simulink model "pi_client"  (R2019b)
settings: Solver=FixedStepAuto  StartTime=0.0  StopTime=10.0  RelTol=1e-3  EnableMultiTasking=on
values from neighbouring files (symbols this model uses):
  B = img(:,:,3)    [pi_client_script.m]
  Blank = R*0    [pi_client_script.m]
  G = img(:,:,2)    [pi_client_script.m]
  R = img(:,:,1)    [pi_client_script.m]
libraries: embdlinuxlib x1, raspberrypilib x1
settings Model: Creator=dhinojosac  LastModifiedBy=dhinojosac
settings SolverCC: PositivePriorityOrder=on
settings OptimizationCC: EnhancedBackFolding=on  PassReuseOutputArgsAs=Individual arguments  ZeroExternalMemoryAtStartup=off  ZeroInternalMemoryAtStartup=off  MaxStackSize=64  OptimizeBlockOrder=speed  DifferentSizesBufferReuse=on  OptimizationCustomize=off  EfficientTunableParamExpr=on
settings DebuggingCC: ParameterTunabilityLossMsg=error
settings HardwareCC: ProdBitPerPointer=32  ProdBitPerSizeT=32  ProdBitPerPtrDiffT=32  ProdLargestAtomicInteger=Long  ProdLargestAtomicFloat=Double  ProdWordSize=32  ProdLongLongMode=on  ProdHWDeviceType=ARM Compatible->ARM Cortex  UseEmbeddedCoderFeatures=off  UseSimulinkCoderFeatures=off
settings RTWCC: SystemTargetFile=ert.tlc  HardwareBoard=Raspberry Pi  TLCOptions="-aInlineSetEventsForThisBaseRateFcn=TLC_FALSE -aSuppressMultiTaskScheduler=TLC_FALSE  -aRateBasedStepFcn=0"  TemplateMakefile=ert_default_tmf  GenerateReport=on  Toolchain=GNU GCC Raspberry Pi  BuildConfiguration=Faster Runs  IncludeHyperlinkInReport=on  LaunchReport=on  GenerateTraceInfo=on  GenerateTraceReport=on  GenerateTraceReportSl=on  GenerateTraceReportSf=on  GenerateTraceReportEml=on
settings CodeAppCC: ForceParamTrailComments=on  IgnoreCustomStorageClasses=off  OperatorAnnotations=on  SimulinkDataObjDesc=on  SFDataObjDesc=on  InsertBlockDesc=on
settings ERTTargetCC: SupportNonInlinedSFcns=on  SupportVariableSizeSignals=on

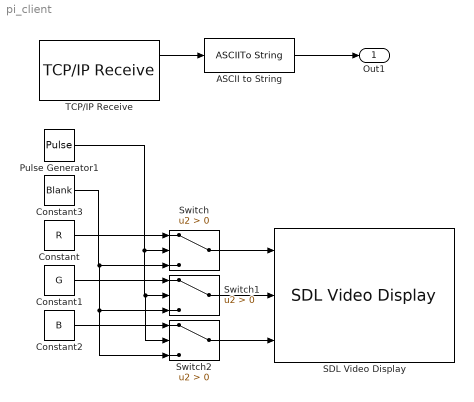
== system pi_client ==
  ASCII to String : ASCIIToString
  Constant : Constant  Value=R  VectorParams1D=off
  Constant1 : Constant  Value=G  VectorParams1D=off
  Constant2 : Constant  Value=B  VectorParams1D=off
  Constant3 : Constant  Value=Blank  VectorParams1D=off
  Pulse Generator1 : DiscretePulseGenerator  PulseType=Time based  Period=10  PulseWidth=5  SampleTime=0.1
  SDL Video Display : embdlinuxlib/SDL Video Display  pixelFormat=RGB  pixelOrder=Planar  rowMajor=on  blockPlatform=Raspberry Pi
      settings: SourceProductName=Simulink Support Package for Raspberry Pi Hardware  SourceProductBaseCode=RASPPI
  Switch : Switch  Criteria=u2 > Threshold
  Switch1 : Switch  Criteria=u2 > Threshold
  Switch2 : Switch  Criteria=u2 > Threshold
  TCP/IP Receive : raspberrypilib/TCP//IP Receive  Mode_=Client  LocalServerPort_=25000  RemoteAddr_=127.0.0.1  RemoteServerPort_=8765  DataType_=uint8  DataSize_=1  SampleTime_=0.1  SimulateUsing=Code generation  ClientPortBindingSelection_=off  ClientPortToBind_=35000  BlockingMode_=off  BlockTimeout_=0.1
      settings: SourceProductName=Simulink Support Package for Raspberry Pi Hardware  SourceProductBaseCode=RASPPI
  Out1 : Outport
  wires:
  TCP/IP Receive/1 -> ASCII to String/1
  ASCII to String/1 -> Out1/1
  Constant1/1 -> Switch1/1
  Constant/1 -> Switch/1
  Constant2/1 -> Switch2/1
  Switch1/1 -> SDL Video Display/2
  Constant3/1 -> Switch1/3, Switch2/3, Switch/3
  Switch/1 -> SDL Video Display/1
  Pulse Generator1/1 -> Switch2/2, Switch1/2, Switch/2
  Switch2/1 -> SDL Video Display/3
